simulink model "TransmissionLineFault"  (R2016b)
settings: Solver=VariableStepAuto  StartTime=0.0  StopTime=10.0  RelTol=1e-3
libraries: powerlib x11, powerlib_meascontrol x2
settings Model: Creator=dj  LastModifiedBy=dj

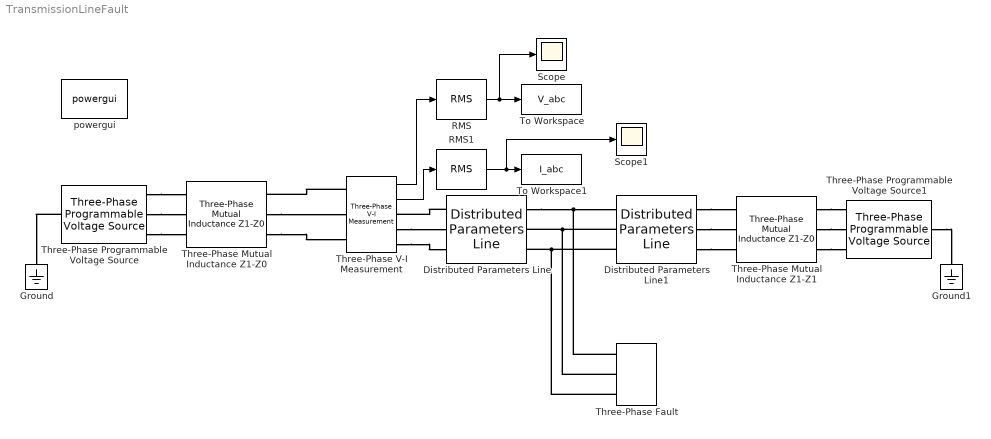
== system TransmissionLineFault ==
  Distributed Parameters Line : powerlib/Elements/Distributed Parameters Line  Phases=3  Frequency=60  Resistance=[0.01273 0.3864]  Inductance="[0.9337e-3  4.1264e-3]"  Capacitance=[12.74e-9 7.751e-9]  Length=100  x1=[7.56052195824063e-13 94.0414085665826 74.7584720367612;376.991118430775 376.991118430775 376.991118430775;2.22282032804376 0.562431876343661 -1.37006811590072]  x2=[4.17739459319107e-12 88.1420635092481 50.8888440939936;376.991118430775 376.991118430775 376.991118430775;2.19051623737059 0.915862922637561 -2.2257297309522]  x3=[2.12996240048792e-14 1.24525169712234 1.40886379577394;376.991118430775 376.991118430775 376.991118430775;0.891674426273457 0.831265474509091 0.855333038571423]  x4=[1.98830894944237e-14 0.602108890060928 1.79029147774271;376.991118430775 376.991118430775 376.991118430775;-2.54632581016302 -2.13107963534388 -2.17064845851155]  x5=0.000565541566995742  V1=[7.561e-13 94.04 74.76;377 377 377;2.223 0.5624 -1.37]  V2=[4.177e-12 88.14 50.89;377 377 377;2.191 0.9159 -2.226]  I1=[2.13e-14 1.245 1.409;377 377 377;0.8917 0.8313 0.8553]  I2=[1.988e-14 0.6021 1.79;377 377 377;-2.546 -2.131 -2.171]  nHarmo=1  Measurements=None
  Distributed Parameters Line1 : powerlib/Elements/Distributed Parameters Line  Phases=3  Frequency=60  Resistance=[0.01273 0.3864]  Inductance="[0.9337e-3  4.1264e-3]"  Capacitance=[12.74e-9 7.751e-9]  Length=100  x1=[4.18635754102815e-12 88.1420635092481 50.8888440939936;376.991118430775 376.991118430775 376.991118430775;2.1913155605001 0.915862922637561 -2.2257297309522]  x2=[8.41072605752851e-13 92.5045631311062 76.6519501798956;376.991118430775 376.991118430775 376.991118430775;2.05476419829754 1.27608654677033 -3.0527638112071]  x3=[1.92516806691056e-14 1.24967585156895 1.41632939557653;376.991118430775 376.991118430775 376.991118430775;-2.51973771381476 0.961414170086409 0.98550872781615]  x4=[2.09690567173597e-14 0.597854099895454 1.78272809465353;376.991118430775 376.991118430775 376.991118430775;0.949315165228293 -2.26119462023257 -2.30081783288978]  x5=0.000565541566995742  V1=[4.186e-12 88.14 50.89;377 377 377;2.191 0.9159 -2.226]  V2=[8.411e-13 92.5 76.65;377 377 377;2.055 1.276 -3.053]  I1=[1.925e-14 1.25 1.416;377 377 377;-2.52 0.9614 0.9855]  I2=[2.097e-14 0.5979 1.783;377 377 377;0.9493 -2.261 -2.301]  nHarmo=1  Measurements=None
  Ground : powerlib/Elements/Ground  LConnTagsString=a
  Ground1 : powerlib/Elements/Ground  LConnTagsString=a
  RMS : powerlib_meascontrol/Measurements/RMS  TrueRMS=on  Freq=60  RMSInit=120  Ts=0
  RMS1 : powerlib_meascontrol/Measurements/RMS  TrueRMS=on  Freq=60  RMSInit=120  Ts=0
  Scope : Scope
  Scope1 : Scope
  Three-Phase Mutual Inductance Z1-Z0 : powerlib/Elements/Three-Phase Mutual Inductance Z1-Z0  LConnTagsString=a|b|c  RConnTagsString=A|B|C  PositiveSequence="[ 2  50e-3]"  ZeroSequence="[4  100e-3]"
  Three-Phase Mutual Inductance Z1-Z1 : powerlib/Elements/Three-Phase Mutual Inductance Z1-Z0  LConnTagsString=a|b|c  RConnTagsString=A|B|C  PositiveSequence="[ 2  50e-3]"  ZeroSequence="[4  100e-3]"
  Three-Phase Programmable Voltage Source : powerlib/Electrical Sources/Three-Phase Programmable Voltage Source  PositiveSequence="[100  0 60]"  VariationEntity=None  VariationType=Table of time-amplitude pairs  VariationTypeAlt=Step  VariationStep=0.5  VariationRate=10  VariationMagnitude=0.3  VariationFrequency=2  VariationTiming=[1 2]  VariationPhaseA=off  Amplitudes=[1 0.8 1.2 1.0]  TimeValues=[0 0.1 0.15 0.2]  HarmonicGeneration=off  HarmonicA=[3 0.2 -25 0]  HarmonicB=[2 0.15 35 2]  Timing="[0.05  3]"  BusType=swing  Pref=0  Qref=0  Qmin=-inf  Qmax=inf
  Three-Phase Programmable Voltage Source1 : powerlib/Electrical Sources/Three-Phase Programmable Voltage Source  PositiveSequence=[100 0 60]  VariationEntity=None  VariationType=Table of time-amplitude pairs  VariationTypeAlt=Step  VariationStep=0.5  VariationRate=10  VariationMagnitude=0.3  VariationFrequency=2  VariationTiming=[1 2]  VariationPhaseA=off  Amplitudes=[1 0.8 1.2 1.0]  TimeValues=[0 0.1 0.15 0.2]  HarmonicGeneration=off  HarmonicA=[3 0.2 -25 0]  HarmonicB=[2 0.15 35 2]  Timing="[0.05  3]"  BusType=swing  Pref=0  Qref=0  Qmin=-inf  Qmax=inf
  Three-Phase V-I Measurement : powerlib/Measurements/Three-Phase V-I Measurement  VoltageMeasurement=phase-to-ground  SetLabelV=off  LabelV=Vabc  Vpu=off  VpuLL=off  CurrentMeasurement=yes  SetLabelI=off  LabelI=Iabc  Ipu=off  Pbase=100e2  Vbase=100  OutputType=Complex  PhasorSimulation=off  PSBequivalent=0
  Three-Phase Fault : powerlib/Elements/Three-Phase Fault  InitialStates=0  FaultA=off  FaultB=off  FaultC=off  GroundFault=off  SwitchTimes="[1/60  5/60]"  External=off  SwitchStatus=NaN  FaultResistance=0.001  GroundResistance=0.01  SnubberResistance=1e6  SnubberCapacitance=inf  Measurements=Fault voltages and currents
  To Workspace : ToWorkspace  VariableName=V_abc  SaveFormat=Timeseries  SampleTime=-1
  To Workspace1 : ToWorkspace  VariableName=I_abc  SaveFormat=Timeseries  SampleTime=-1
  powergui : powerlib/powergui  Priority=1  SimulationMode=Continuous  SolverType=Tustin/Backward Euler (TBE)  SampleTime=50e-6  frequency=60  SPID=off  DisableSnubberDevices=off  DisableRonSwitches=off  DisableVfSwitches=off  SwTol=0  DisplayEquations=off  Interpol=off  ExternalGateDelay=off  methode=off  Ts=10  FunctionMessages=off  echomessages=off  HookPort=off  EnableUseOfTLC=off  x0status=blocks  frequencyindice=0  Pbase=100e6  ErrMax=1e-4  Iterations=50  UnitsV=kV  UnitsW=MW  buscounter=0  RestoreLinks=warning  ResistiveCurrentMeasurement=off  Frange=[0:2:500]  Ylog=off  Xlog=on  ShowGrid=off  save=off  variable=ZData  structure=0  ZoomFFT=off  StartTime=0.0  cycles=1  DisplayStyle=1  fundamental=60  FreqAxis=off  MaxFrequency=1000  frequencyindicesteady=1  RmsSteady=1  display=off
  wires:
  Three-Phase V-I Measurement/1 -> RMS/1
  RMS/1 -> Scope/1, To Workspace/1
  RMS1/1 -> Scope1/1, To Workspace1/1
  Three-Phase V-I Measurement/2 -> RMS1/1
  connections:
  Three-Phase Programmable Voltage Source/LConn1 -- Ground/LConn1
  Three-Phase Programmable Voltage Source/RConn1 -- Three-Phase Mutual Inductance Z1-Z0/LConn1
  Three-Phase Programmable Voltage Source/RConn2 -- Three-Phase Mutual Inductance Z1-Z0/LConn2
  Three-Phase Programmable Voltage Source/RConn3 -- Three-Phase Mutual Inductance Z1-Z0/LConn3
  Three-Phase Mutual Inductance Z1-Z1/RConn1 -- Three-Phase Programmable Voltage Source1/RConn3
  Three-Phase Mutual Inductance Z1-Z1/RConn2 -- Three-Phase Programmable Voltage Source1/RConn2
  Three-Phase Mutual Inductance Z1-Z1/RConn3 -- Three-Phase Programmable Voltage Source1/RConn1
  Three-Phase Programmable Voltage Source1/LConn1 -- Ground1/LConn1
  Three-Phase V-I Measurement/LConn1 -- Three-Phase Mutual Inductance Z1-Z0/RConn1
  Three-Phase Mutual Inductance Z1-Z0/RConn2 -- Three-Phase V-I Measurement/LConn2
  Three-Phase Mutual Inductance Z1-Z0/RConn3 -- Three-Phase V-I Measurement/LConn3
  Distributed Parameters Line/LConn1 -- Three-Phase V-I Measurement/RConn1
  Three-Phase V-I Measurement/RConn2 -- Distributed Parameters Line/LConn2
  Three-Phase V-I Measurement/RConn3 -- Distributed Parameters Line/LConn3
  Distributed Parameters Line1/RConn1 -- Three-Phase Mutual Inductance Z1-Z1/LConn1
  Distributed Parameters Line1/RConn2 -- Three-Phase Mutual Inductance Z1-Z1/LConn2
  Distributed Parameters Line1/RConn3 -- Three-Phase Mutual Inductance Z1-Z1/LConn3
  Distributed Parameters Line/RConn1 -- Three-Phase Fault/LConn1 -- Distributed Parameters Line1/LConn1
  Distributed Parameters Line1/LConn2 -- Three-Phase Fault/LConn2 -- Distributed Parameters Line/RConn2
  Distributed Parameters Line1/LConn3 -- Three-Phase Fault/LConn3 -- Distributed Parameters Line/RConn3
